simulink model "BasicModelTarget"  (Simulink 7.5)
settings: Solver=ode5  StartTime=0.0  StopTime=inf  FixedStep=sp/2  RelTol=1e-3
undefined symbols (not defined in the file or in its folder): AAz, BBz, sp
libraries: xpcnilib x10, xpclib x7
CloseFcn:
  | rtwprivate ssgencode ModelCloseRequest readecnoder
settings Model: Creator=Justin  LastModifiedBy=Justin  ExtModeArmWhenConnect=off  BufferReuse=off
settings DataIOCC: LimitDataPoints=off  MaxDataPoints=10000  SignalLoggingName=sigsOut
settings OptimizationCC: BlockReduction=off  BooleanDataType=off  OptimizeBlockIOStorage=off  BufferReuse=off  EnforceIntegerDowncast=off  ExpressionFolding=off  FoldNonRolledExpr=off  LocalBlockOutputs=off  InitFltsAndDblsToZero=on
settings DebuggingCC: SaveWithParameterizedLinksMsg=none  SignalResolutionControl=TryResolveAllWithWarning  SolverPrmCheckMsg=none  MultiTaskDSMMsg=warning  MultiTaskCondExecSysMsg=none  StrictBusMsg=None
settings HardwareCC: ProdIntDivRoundTo=Zero  ProdEndianess=LittleEndian  ProdHWDeviceType=Generic->32-bit x86 compatible  TargetHWDeviceType=32-bit Generic
settings RTWCC: SystemTargetFile=xpctarget.tlc  TemplateMakefile=xpc_default_tmf  Description=xPC Target  ProcessScript=xpctarget_make_rtw_hook  IncludeERTFirstTime=on  RTWCompilerOptimization=On
settings xpcTargetCC: TargetFcnLib=ansi_tfl_tmw.mat  TargetFunctionLibrary=ANSI_C  ERTCodeCoverageTool=None  ParMdlRefBuildCompliant=off  PortableWordSizes=off  xPCLoadParamSetFile=off

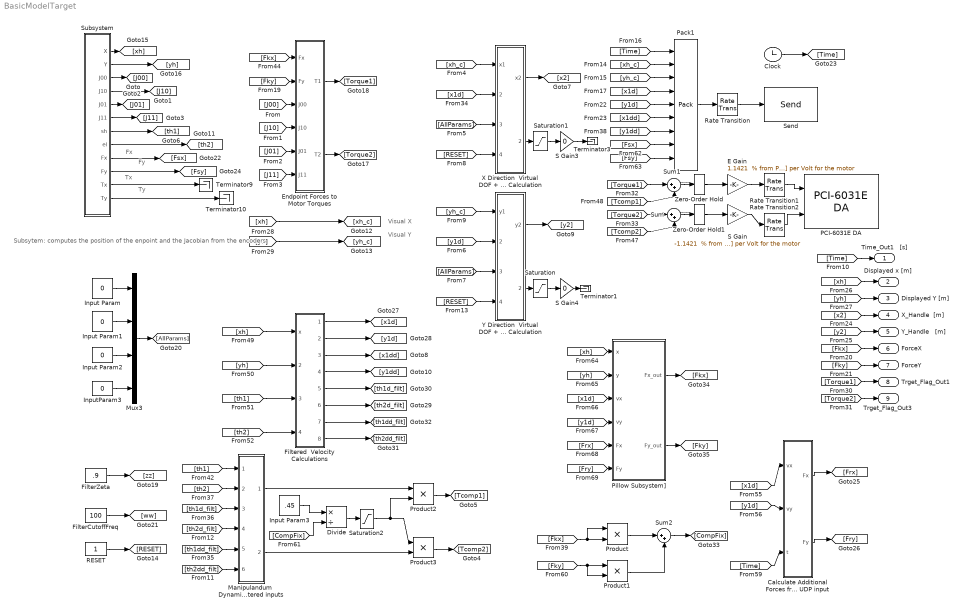
== system BasicModelTarget ==
  note: Subsytem:
      |  computes the position of the
      | enpoint and the Jacobian from
      | the encoders
  note: Ty
  note: Tx
  note: Fy
  note: Fx
  note: Visual X
  note: Visual Y
  " Calculate Additional Forces from UDP input" : Subsystem
  " Pillow Subsystem]" : Subsystem
  Clock : Clock
      settings: Decimation=10
  Divide : Product  Inputs=*/  OutDataType=fixdt(1, 16)  OutScaling=2^-10
  E Gain : Gain  Gain="1.1421  % from PCIO.H: [Nm] per Volt for the motor"  ParameterDataType=sfix(16)  ParameterScaling=2^0  OutDataType=sfix(16)  OutScaling=2^0  SaturateOnIntegerOverflow=on  OutDataTypeStr=Inherit: Same as input  ParamDataTypeStr=Inherit: Same as input
  Endpoint Forces to Motor Torques : Subsystem
  FilterCutoffFreq : Constant  Value=100  OutDataType=sfix(16)  OutScaling=2^0
  FilterZeta : Constant  Value=.9  OutDataType=sfix(16)  OutScaling=2^0
  Filtered  Velocity Calculations : Subsystem
  Input Param : Constant  Value=0  OutDataType=sfix(16)  OutScaling=2^0
  Input Param1 : Constant  Value=0  OutDataType=sfix(16)  OutScaling=2^0
  Input Param2 : Constant  Value=0  OutDataType=sfix(16)  OutScaling=2^0
  Input Param3 : Constant  Value=.45  OutDataType=sfix(16)  OutScaling=2^0
  InputParam3 : Constant  Value=0  OutDataType=sfix(16)  OutScaling=2^0
  Manipulandum  Dynamic Compensation: will function poorly with unfiltered inputs : Subsystem
  Mux3 : Mux
  PCI-6031E DA : xpcnilib/D//A/E Series/PCI-6031E DA  channel=[1 2]  range=[-10 -10]  reset=[1]  initValue=[0]  sampletime=sp  slot=-1
  Pack1 : xpclib/UDP/Pack  datatypes={'double','double','double','double','double','double','double','double','double'}  byteAlign=1
  Product{,1..3} (4 alike) : Product  OutDataType=fixdt(1, 16)  OutScaling=2^0  RndMeth=Zero
  RESET : Constant  OutDataType=sfix(16)  OutScaling=2^0
  Rate Transition : RateTransition
  Rate Transition1 : RateTransition
  Rate Transition2 : RateTransition
  S Gain : Gain  Gain="-1.1421  % from PCIO.H: [Nm] per Volt for the motor"  ParameterDataType=sfix(16)  ParameterScaling=2^0  OutDataType=sfix(16)  OutScaling=2^0  SaturateOnIntegerOverflow=on  OutDataTypeStr=Inherit: Same as input  ParamDataTypeStr=Inherit: Same as input
  S Gain3 : Gain  Gain=0  ParameterDataType=sfix(16)  ParameterScaling=2^0  OutDataType=sfix(16)  OutScaling=2^0  SaturateOnIntegerOverflow=on  OutDataTypeStr=Inherit: Same as input  ParamDataTypeStr=Inherit: Same as input
  S Gain4 : Gain  Gain=0  ParameterDataType=sfix(16)  ParameterScaling=2^0  OutDataType=sfix(16)  OutScaling=2^0  SaturateOnIntegerOverflow=on  OutDataTypeStr=Inherit: Same as input  ParamDataTypeStr=Inherit: Same as input
  Saturation : Saturate  UpperLimit=20  LowerLimit=-20
  Saturation1 : Saturate  UpperLimit=20  LowerLimit=-20
  Saturation2 : Saturate  UpperLimit=.4  LowerLimit=0
  Send : xpclib/UDP/Send  ipAddress=192.168.0.1  ipPort=25000  localPort=-1  vblLen=off  sampletime=sp*5
  Subsystem : Subsystem
  Sum : Sum  Inputs=|++  OutDataType=sfix(16)  OutScaling=2^0
  Sum1 : Sum  Inputs=|++  OutDataType=sfix(16)  OutScaling=2^0
  Sum2 : Sum  Inputs=|++  OutDataType=fixdt(1, 16)  OutScaling=2^0
  Terminator{1,3,9..10} (4 alike) : Terminator
  "X Direction  Virtual DOF + Endpoint Force Calculation " : Subsystem
  Y Direction  Virtual DOF + Endpoint Force Calculation : Subsystem
  Zero-Order Hold : ZeroOrderHold  SampleTime=sp*2
  Zero-Order Hold1 : ZeroOrderHold  SampleTime=sp*2
  Time_Out1   [s] : Outport  OutDataType=sfix(16)  OutScaling=2^0
  Displayed x [m] : Outport  Port=2  OutDataType=sfix(16)  OutScaling=2^0
  Displayed Y [m] : Outport  Port=3  OutDataType=sfix(16)  OutScaling=2^0
  X_Handle  [m] : Outport  Port=4  OutDataType=sfix(16)  OutScaling=2^0
  Y_Handle   [m] : Outport  Port=5  OutDataType=sfix(16)  OutScaling=2^0
  ForceX : Outport  Port=6  OutDataType=sfix(16)  OutScaling=2^0
  ForceY : Outport  Port=7  OutDataType=sfix(16)  OutScaling=2^0
  Trget_Flag_Out1 : Outport  Port=8  OutDataType=sfix(16)  OutScaling=2^0
  Trget_Flag_Out3 : Outport  Port=9  OutDataType=sfix(16)  OutScaling=2^0
  wires:
  Pack1/1 -> Rate Transition/1
  Clock/1 -> [Time]
  Subsystem/12(Ty) -> Terminator10/1
  Subsystem/11(Tx) -> Terminator9/1
  Subsystem/8(el) -> [th2]
  Subsystem/7(sh) -> [th1]
  E Gain/1 -> Rate Transition1/1
  S Gain/1 -> Rate Transition2/1
  Subsystem/10(Fy) -> [Fsy]
  [x2] -> X_Handle  [m]/1
  [xh] -> [xh_c]
  [yh] -> [yh_c]
  [y2] -> Y_Handle   [m]/1
  [Torque1] -> Trget_Flag_Out1/1
  [Torque2] -> Trget_Flag_Out3/1
  [Fkx] -> ForceX/1
  [Fky] -> ForceY/1
  [xh] -> Displayed x [m]/1
  [yh] -> Displayed Y [m]/1
  [Fky] -> Endpoint Forces to Motor Torques/2(Fy)
  [J00] -> Endpoint Forces to Motor Torques/3(J00)
  [J10] -> Endpoint Forces to Motor Torques/4(J10)
  [J01] -> Endpoint Forces to Motor Torques/5(J01)
  [J11] -> Endpoint Forces to Motor Torques/6(J11)
  Endpoint Forces to Motor Torques/1(T1) -> [Torque1]
  Endpoint Forces to Motor Torques/2(T2) -> [Torque2]
  [yh_c] -> Pack1/3
  [x1d] -> Pack1/4
  [y1d] -> Pack1/5
  [x1dd] -> Pack1/6
  "X Direction  Virtual DOF + Endpoint Force Calculation "/1(x2) -> [x2]
  [AllParams] -> "X Direction  Virtual DOF + Endpoint Force Calculation "/3(Params)
  [xh_c] -> "X Direction  Virtual DOF + Endpoint Force Calculation "/1(x1)
  Y Direction  Virtual DOF + Endpoint Force Calculation/2(Fky) -> Saturation/1
  Y Direction  Virtual DOF + Endpoint Force Calculation/1(y2) -> [y2]
  [RESET] -> Y Direction  Virtual DOF + Endpoint Force Calculation/4(Reset)
  [yh_c] -> Y Direction  Virtual DOF + Endpoint Force Calculation/1(y1)
  "X Direction  Virtual DOF + Endpoint Force Calculation "/2(Fkx) -> Saturation1/1
  Saturation1/1 -> S Gain3/1
  [y1dd] -> Pack1/7
  [x1d] -> "X Direction  Virtual DOF + Endpoint Force Calculation "/2(x1d)
  [RESET] -> "X Direction  Virtual DOF + Endpoint Force Calculation "/4(Reset)
  Mux3/1 -> [AllParams]
  Input Param/1 -> Mux3/1
  Input Param1/1 -> Mux3/2
  Input Param2/1 -> Mux3/3
  InputParam3/1 -> Mux3/4
  [y1d] -> Y Direction  Virtual DOF + Endpoint Force Calculation/2(y1d)
  [AllParams] -> Y Direction  Virtual DOF + Endpoint Force Calculation/3(Params)
  Subsystem/1(X) -> [xh]
  Subsystem/2(Y) -> [yh]
  Subsystem/3(J00) -> [J00]
  Subsystem/4(J10) -> [J10]
  Subsystem/5(J01) -> [J01]
  Subsystem/6(J11) -> [J11]
  [Time] -> Time_Out1   [s]/1
  [th1] -> Manipulandum  Dynamic Compensation: will function poorly with unfiltered inputs/1(th1)
  [th2] -> Manipulandum  Dynamic Compensation: will function poorly with unfiltered inputs/2(th2)
  [th1d_filt] -> Manipulandum  Dynamic Compensation: will function poorly with unfiltered inputs/3(th1d)
  [th2d_filt] -> Manipulandum  Dynamic Compensation: will function poorly with unfiltered inputs/4(th2d)
  [th1dd_filt] -> Manipulandum  Dynamic Compensation: will function poorly with unfiltered inputs/5(th1dd)
  [th2dd_filt] -> Manipulandum  Dynamic Compensation: will function poorly with unfiltered inputs/6(th2dd)
  [Torque2] -> Sum/1
  [Tcomp2] -> Sum/2
  Sum/1 -> Zero-Order Hold1/1
  [Tcomp1] -> Sum1/2
  [Torque1] -> Sum1/1
  Sum1/1 -> Zero-Order Hold/1
  Saturation/1 -> S Gain4/1
  Subsystem/9(Fx) -> [Fsx]
  Zero-Order Hold/1 -> E Gain/1
  Zero-Order Hold1/1 -> S Gain/1
  FilterZeta/1 -> [zz]
  FilterCutoffFreq/1 -> [ww]
  RESET/1 -> [RESET]
  S Gain4/1 -> Terminator1/1
  S Gain3/1 -> Terminator3/1
  Rate Transition/1 -> Send/1
  Rate Transition1/1 -> PCI-6031E DA/1
  Rate Transition2/1 -> PCI-6031E DA/2
  [Fkx] -> Endpoint Forces to Motor Torques/1(Fx)
  [Time] -> Pack1/1
  [xh_c] -> Pack1/2
  [Fkx] -> Product/1, Product/2
  [Fky] -> Product1/1, Product1/2
  Product/1 -> Sum2/1
  Product1/1 -> Sum2/2
  Manipulandum  Dynamic Compensation: will function poorly with unfiltered inputs/1(Tc1) -> Product2/1
  Manipulandum  Dynamic Compensation: will function poorly with unfiltered inputs/2(Tc2) -> Product3/2
  Product3/1 -> [Tcomp2]
  Product2/1 -> [Tcomp1]
  Input Param3/1 -> Divide/1
  [CompFix] -> Divide/2
  Divide/1 -> Saturation2/1
  Saturation2/1 -> Product2/2, Product3/1
  Sum2/1 -> [CompFix]
  [Fsx] -> Pack1/8
  [Fsy] -> Pack1/9
  [xh] -> " Pillow Subsystem]"/1(x)
  [yh] -> " Pillow Subsystem]"/2(y)
  [x1d] -> " Pillow Subsystem]"/3(vx)
  [y1d] -> " Pillow Subsystem]"/4(vy)
  [Frx] -> " Pillow Subsystem]"/5(Fx)
  [Fry] -> " Pillow Subsystem]"/6(Fy)
  " Pillow Subsystem]"/1(Fx_out) -> [Fkx]
  " Pillow Subsystem]"/2(Fy_out) -> [Fky]
  Filtered  Velocity Calculations/1(Out1) -> [x1d]
  Filtered  Velocity Calculations/2(Out2) -> [y1d]
  [xh] -> Filtered  Velocity Calculations/1(x)
  [yh] -> Filtered  Velocity Calculations/2(In2)
  [th1] -> Filtered  Velocity Calculations/3(In3)
  [th2] -> Filtered  Velocity Calculations/4(In4)
  Filtered  Velocity Calculations/3(xdd) -> [x1dd]
  Filtered  Velocity Calculations/4(Out4) -> [y1dd]
  Filtered  Velocity Calculations/5(Out5) -> [th1d_filt]
  Filtered  Velocity Calculations/6(Out6) -> [th2d_filt]
  Filtered  Velocity Calculations/7(Out7) -> [th1dd_filt]
  Filtered  Velocity Calculations/8(Out8) -> [th2dd_filt]
  [x1d] -> " Calculate Additional Forces from UDP input"/1(vx)
  [y1d] -> " Calculate Additional Forces from UDP input"/2(vy)
  " Calculate Additional Forces from UDP input"/1(Fx) -> [Frx]
  " Calculate Additional Forces from UDP input"/2(Fy) -> [Fry]
  [Time] -> " Calculate Additional Forces from UDP input"/3(t)

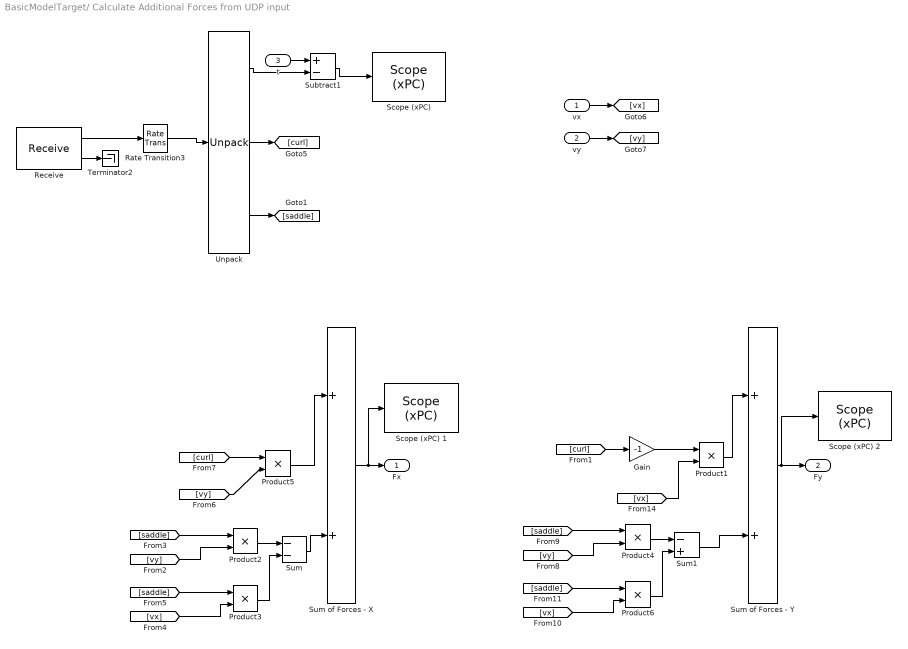
== system BasicModelTarget/ Calculate Additional Forces from UDP input ==
  vx : Inport  OutDataType=fixdt(1, 16)  OutScaling=2^0
  vy : Inport  Port=2  OutDataType=fixdt(1, 16)  OutScaling=2^0
  t : Inport  Port=3  OutDataType=fixdt(1, 16)  OutScaling=2^0
  Gain : Gain  Gain=-1  ParameterDataType=fixdt(1, 16)  ParameterScaling=2^0  OutDataType=fixdt(1, 16)  OutScaling=2^0
  Product{1..6} (6 alike) : Product  OutDataType=fixdt(1, 16)  OutScaling=2^0  RndMeth=Zero
  Rate Transition3 : RateTransition
  Receive : xpclib/UDP/Receive  ipAddress=0.0.0.0  ipPort=25000  width=8*3  vblLen=off  sampletime=sp*5
  "Scope (xPC) " : xpclib/Misc./Scope (xPC)   SystemSampleTime=-1  scopeno=4  scopetype=Target  autostart=on  viewmode=Numerical  formatstr='%15.6f'  grid=on  ylimits=[-6,6]  nosamples=250  noprepostsamples=0  interleave=1  triggermode=FreeRun  triggersignal=1  triggerlevel=0.0  triggerslope=Either  triggerscope=1  triggersample=0  filename=data.dat  mode=Lazy  writesize=512  autorestart=off  dynamicfilemode=off  maxwritefilesize=512*1024^2
  Scope (xPC) 1 : xpclib/Misc./Scope (xPC)   SystemSampleTime=-1  scopeno=1  scopetype=Target  autostart=on  viewmode=Graphical redraw  formatstr='%15.6f'  grid=on  ylimits=[-6,6]  nosamples=250  noprepostsamples=0  interleave=1  triggermode=FreeRun  triggersignal=1  triggerlevel=0.0  triggerslope=Either  triggerscope=1  triggersample=0  filename=data.dat  mode=Lazy  writesize=512  autorestart=off  dynamicfilemode=off  maxwritefilesize=512*1024^2
  Scope (xPC) 2 : xpclib/Misc./Scope (xPC)   SystemSampleTime=-1  scopeno=2  scopetype=Target  autostart=on  viewmode=Graphical redraw  formatstr='%15.6f'  grid=on  ylimits=[-6,6]  nosamples=250  noprepostsamples=0  interleave=1  triggermode=FreeRun  triggersignal=1  triggerlevel=0.0  triggerslope=Either  triggerscope=1  triggersample=0  filename=data.dat  mode=Lazy  writesize=512  autorestart=off  dynamicfilemode=off  maxwritefilesize=512*1024^2
  Subtract1 : Sum  Inputs=+-  OutDataType=fixdt(1, 16)  OutScaling=2^-10
  Sum : Sum  Inputs=--  OutDataType=fixdt(1, 16)  OutScaling=2^-10
  Sum of Forces - X : Sum  OutDataType=fixdt(1, 16)  OutScaling=2^-10
  Sum of Forces - Y : Sum  OutDataType=fixdt(1, 16)  OutScaling=2^-10
  Sum1 : Sum  Inputs=-+  OutDataType=fixdt(1, 16)  OutScaling=2^-10
  Terminator2 : Terminator
  Unpack : xpclib/UDP/Unpack  dimensions={1,1,1}  datatypes={'double','double','double'}  byteAlign=1
  Fx : Outport  OutDataType=fixdt(1, 16)  OutScaling=2^0
  Fy : Outport  Port=2  OutDataType=fixdt(1, 16)  OutScaling=2^0
  wires:
  Sum1/1 -> Sum of Forces - Y/2
  [vy] -> Product4/2
  Product6/1 -> Sum1/2
  [vx] -> Product6/2
  [saddle] -> Product6/1
  Product4/1 -> Sum1/1
  [saddle] -> Product4/1
  [vy] -> Product2/2
  Product3/1 -> Sum/2
  [vx] -> Product3/2
  [saddle] -> Product3/1
  Sum/1 -> Sum of Forces - X/2
  Product2/1 -> Sum/1
  [saddle] -> Product2/1
  Unpack/3 -> [saddle]
  Product1/1 -> Sum of Forces - Y/1
  [curl] -> Gain/1
  Gain/1 -> Product1/1
  [vx] -> Product1/2
  Product5/1 -> Sum of Forces - X/1
  Unpack/2 -> [curl]
  Unpack/1 -> Subtract1/2
  Sum of Forces - Y/1 -> Scope (xPC) 2/1, Fy/1
  [vy] -> Product5/2
  [curl] -> Product5/1
  vy/1 -> [vy]
  vx/1 -> [vx]
  Sum of Forces - X/1 -> Scope (xPC) 1/1, Fx/1
  t/1 -> Subtract1/1
  Rate Transition3/1 -> Unpack/1
  Receive/1 -> Rate Transition3/1
  Subtract1/1 -> "Scope (xPC) "/1
  Receive/2 -> Terminator2/1

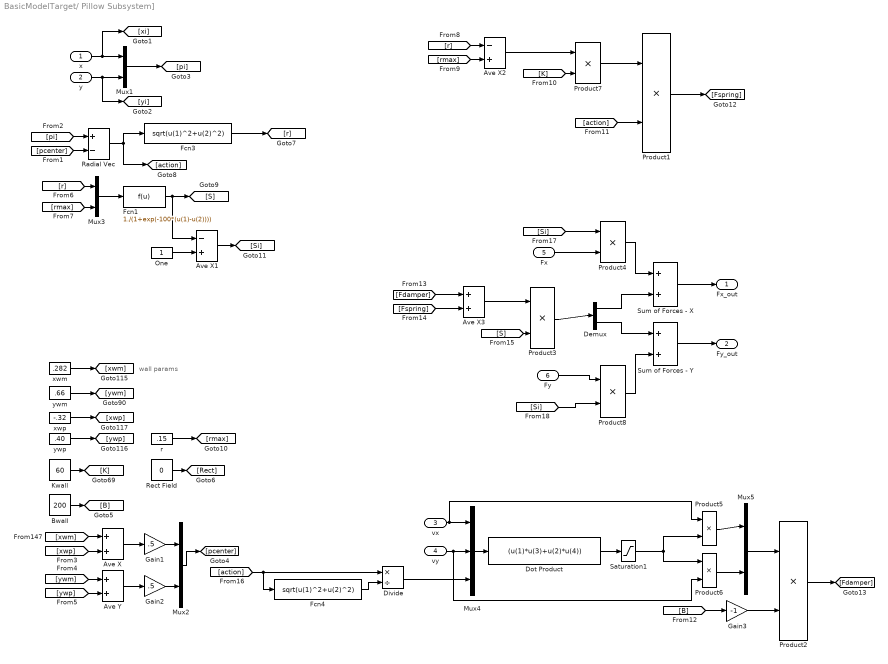
== system BasicModelTarget/ Pillow Subsystem] ==
  note: wall params
  x : Inport  OutDataType=fixdt(1, 16)  OutScaling=2^0
  y : Inport  Port=2  OutDataType=fixdt(1, 16)  OutScaling=2^0
  vx : Inport  Port=3  OutDataType=fixdt(1, 16)  OutScaling=2^0
  vy : Inport  Port=4  OutDataType=fixdt(1, 16)  OutScaling=2^0
  Fx : Inport  Port=5  OutDataType=fixdt(1, 16)  OutScaling=2^0
  Fy : Inport  Port=6  OutDataType=fixdt(1, 16)  OutScaling=2^0
  Ave X : Sum  OutDataType=fixdt(1, 16)  OutScaling=2^-10
  Ave X1 : Sum  Inputs=-+  OutDataType=fixdt(1, 16)  OutScaling=2^-10
  Ave X2 : Sum  Inputs=-+  OutDataType=fixdt(1, 16)  OutScaling=2^-10
  Ave X3 : Sum  OutDataType=fixdt(1, 16)  OutScaling=2^-10
  Ave Y : Sum  OutDataType=fixdt(1, 16)  OutScaling=2^-10
  Bwall : Constant  Value=200  OutDataType=sfix(16)  OutScaling=2^0
  Demux : Demux  Outputs=2
  Divide : Product  Inputs=*/  OutDataType=fixdt(1, 16)  OutScaling=2^-10
  Dot Product : Fcn  Expr=(u(1)*u(3)+u(2)*u(4))
  Fcn1 : Fcn  Expr=1./(1+exp(-100*(u(1)-u(2))))
  Fcn3 : Fcn  Expr=sqrt(u(1)^2+u(2)^2)
  Fcn4 : Fcn  Expr=sqrt(u(1)^2+u(2)^2)
  Gain1 : Gain  Gain=.5  ParameterDataType=fixdt(1, 16)  ParameterScaling=2^0  OutDataType=fixdt(1, 16)  OutScaling=2^0
  Gain2 : Gain  Gain=.5  ParameterDataType=fixdt(1, 16)  ParameterScaling=2^0  OutDataType=fixdt(1, 16)  OutScaling=2^0
  Gain3 : Gain  Gain=-1  ParameterDataType=fixdt(1, 16)  ParameterScaling=2^0  OutDataType=fixdt(1, 16)  OutScaling=2^0
  Kwall : Constant  Value=60  OutDataType=sfix(16)  OutScaling=2^0
  Mux{1..3,5} (4 alike) : Mux  Inputs=2
  Mux4 : Mux  Inputs=3
  One : Constant  OutDataType=sfix(16)  OutScaling=2^0
  Product{1..8} (8 alike) : Product  OutDataType=sfix(16)  OutScaling=2^0  RndMeth=Zero
  Radial Vec : Sum  Inputs=+-  OutDataType=fixdt(1, 16)  OutScaling=2^-10
  Rect Field : Constant  Value=0  OutDataType=sfix(16)  OutScaling=2^0
  Saturation1 : Saturate  UpperLimit=inf  LowerLimit=0
  Sum of Forces - X : Sum  OutDataType=fixdt(1, 16)  OutScaling=2^-10
  Sum of Forces - Y : Sum  OutDataType=fixdt(1, 16)  OutScaling=2^-10
  r : Constant  Value=.15  OutDataType=sfix(16)  OutScaling=2^0
  xwm : Constant  Value=.282  OutDataType=sfix(16)  OutScaling=2^0
  xwp : Constant  Value=-.32  OutDataType=sfix(16)  OutScaling=2^0
  ywm : Constant  Value=.66  OutDataType=sfix(16)  OutScaling=2^0
  ywp : Constant  Value=.40  OutDataType=sfix(16)  OutScaling=2^0
  Fx_out : Outport  OutDataType=fixdt(1, 16)  OutScaling=2^0
  Fy_out : Outport  Port=2  OutDataType=fixdt(1, 16)  OutScaling=2^0
  wires:
  ywp/1 -> [ywp]
  xwp/1 -> [xwp]
  xwm/1 -> [xwm]
  ywm/1 -> [ywm]
  Kwall/1 -> [K]
  Sum of Forces - X/1 -> Fx_out/1
  Sum of Forces - Y/1 -> Fy_out/1
  x/1 -> Mux1/1, [xi]
  y/1 -> Mux1/2, [yi]
  Mux1/1 -> [pi]
  Mux2/1 -> [pcenter]
  [xwm] -> Ave X/1
  [xwp] -> Ave X/2
  [ywp] -> Ave Y/2
  [ywm] -> Ave Y/1
  Ave X/1 -> Gain1/1
  Gain1/1 -> Mux2/1
  Ave Y/1 -> Gain2/1
  Gain2/1 -> Mux2/2
  Bwall/1 -> [B]
  Rect Field/1 -> [Rect]
  [pi] -> Radial Vec/1
  [pcenter] -> Radial Vec/2
  Radial Vec/1 -> Fcn3/1, [action]
  Fcn3/1 -> [r]
  r/1 -> [rmax]
  [r] -> Mux3/1
  [rmax] -> Mux3/2
  Mux3/1 -> Fcn1/1
  Fcn1/1 -> Ave X1/1, [S]
  One/1 -> Ave X1/2
  Ave X1/1 -> [Si]
  [r] -> Ave X2/1
  [rmax] -> Ave X2/2
  Ave X2/1 -> Product7/1
  [K] -> Product7/2
  Product7/1 -> Product1/1
  [action] -> Product1/2
  Product1/1 -> [Fspring]
  vx/1 -> Mux4/1, Product5/1
  vy/1 -> Mux4/2, Product6/2
  Product2/1 -> [Fdamper]
  [Fdamper] -> Ave X3/1
  [Fspring] -> Ave X3/2
  Ave X3/1 -> Product3/1
  [S] -> Product3/2
  Product3/1 -> Demux/1
  Product4/1 -> Sum of Forces - X/1
  Demux/1 -> Sum of Forces - X/2
  Demux/2 -> Sum of Forces - Y/1
  Fy/1 -> Product8/1
  [Si] -> Product4/1
  Fx/1 -> Product4/2
  Mux4/1 -> Dot Product/1
  Mux5/1 -> Product2/1
  [action] -> Fcn4/1, Divide/1
  Divide/1 -> Mux4/3
  Fcn4/1 -> Divide/2
  [B] -> Gain3/1
  Gain3/1 -> Product2/2
  Dot Product/1 -> Saturation1/1
  Product5/1 -> Mux5/1
  Product6/1 -> Mux5/2
  Saturation1/1 -> Product5/2, Product6/1
  [Si] -> Product8/2
  Product8/1 -> Sum of Forces - Y/2

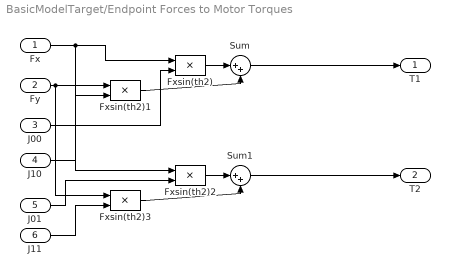
== system BasicModelTarget/Endpoint Forces to Motor Torques ==
  Fx : Inport  OutDataType=sfix(16)  OutScaling=2^0
  Fy : Inport  Port=2  OutDataType=sfix(16)  OutScaling=2^0
  J00 : Inport  Port=3  OutDataType=sfix(16)  OutScaling=2^0
  J10 : Inport  Port=4  OutDataType=sfix(16)  OutScaling=2^0
  J01 : Inport  Port=5  OutDataType=sfix(16)  OutScaling=2^0
  J11 : Inport  Port=6  OutDataType=sfix(16)  OutScaling=2^0
  Fxsin(th2){,1..3} (4 alike) : Product  OutDataType=sfix(16)  OutScaling=2^0  SaturateOnIntegerOverflow=on  OutDataTypeStr=Inherit: Same as first input
  Sum : Sum  Inputs=|++  OutDataType=sfix(16)  OutScaling=2^0  SaturateOnIntegerOverflow=on  InputSameDT=on  OutDataTypeStr=Inherit: Same as first input
  Sum1 : Sum  Inputs=|++  OutDataType=sfix(16)  OutScaling=2^0  SaturateOnIntegerOverflow=on  InputSameDT=on  OutDataTypeStr=Inherit: Same as first input
  T1 : Outport  OutDataType=sfix(16)  OutScaling=2^0
  T2 : Outport  Port=2  OutDataType=sfix(16)  OutScaling=2^0
  wires:
  Sum/1 -> T1/1
  Fxsin(th2)/1 -> Sum/1
  Fxsin(th2)1/1 -> Sum/2
  Fxsin(th2)2/1 -> Sum1/1
  Fxsin(th2)3/1 -> Sum1/2
  Sum1/1 -> T2/1
  Fx/1 -> Fxsin(th2)/1, Fxsin(th2)2/1
  Fy/1 -> Fxsin(th2)1/1, Fxsin(th2)3/1
  J11/1 -> Fxsin(th2)3/2
  J01/1 -> Fxsin(th2)2/2
  J10/1 -> Fxsin(th2)1/2
  J00/1 -> Fxsin(th2)/2

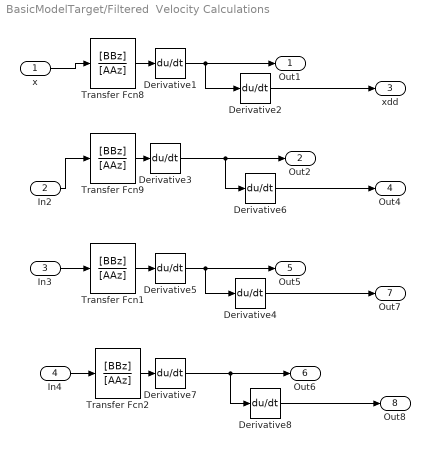
== system BasicModelTarget/Filtered  Velocity Calculations ==
  x : Inport  OutDataType=sfix(16)  OutScaling=2^0
  In2 : Inport  Port=2  OutDataType=sfix(16)  OutScaling=2^0
  In3 : Inport  Port=3  OutDataType=sfix(16)  OutScaling=2^0
  In4 : Inport  Port=4  OutDataType=sfix(16)  OutScaling=2^0
  Derivative{1..8} (8 alike) : Derivative
  Transfer Fcn{1..2,8..9} (4 alike) : TransferFcn  Numerator=[BBz]  Denominator=[AAz]
  Out1 : Outport  OutDataType=sfix(16)  OutScaling=2^0
  Out2 : Outport  Port=2  OutDataType=sfix(16)  OutScaling=2^0
  xdd : Outport  Port=3  OutDataType=sfix(16)  OutScaling=2^0
  Out4 : Outport  Port=4  OutDataType=sfix(16)  OutScaling=2^0
  Out5 : Outport  Port=5  OutDataType=sfix(16)  OutScaling=2^0
  Out6 : Outport  Port=6  OutDataType=sfix(16)  OutScaling=2^0
  Out7 : Outport  Port=7  OutDataType=sfix(16)  OutScaling=2^0
  Out8 : Outport  Port=8  OutDataType=sfix(16)  OutScaling=2^0
  wires:
  x/1 -> Transfer Fcn8/1
  Derivative1/1 -> Out1/1, Derivative2/1
  Derivative3/1 -> Out2/1, Derivative6/1
  In2/1 -> Transfer Fcn9/1
  Transfer Fcn8/1 -> Derivative1/1
  Transfer Fcn9/1 -> Derivative3/1
  In3/1 -> Transfer Fcn1/1
  In4/1 -> Transfer Fcn2/1
  Derivative2/1 -> xdd/1
  Derivative6/1 -> Out4/1
  Derivative5/1 -> Out5/1, Derivative4/1
  Derivative7/1 -> Out6/1, Derivative8/1
  Transfer Fcn1/1 -> Derivative5/1
  Transfer Fcn2/1 -> Derivative7/1
  Derivative4/1 -> Out7/1
  Derivative8/1 -> Out8/1

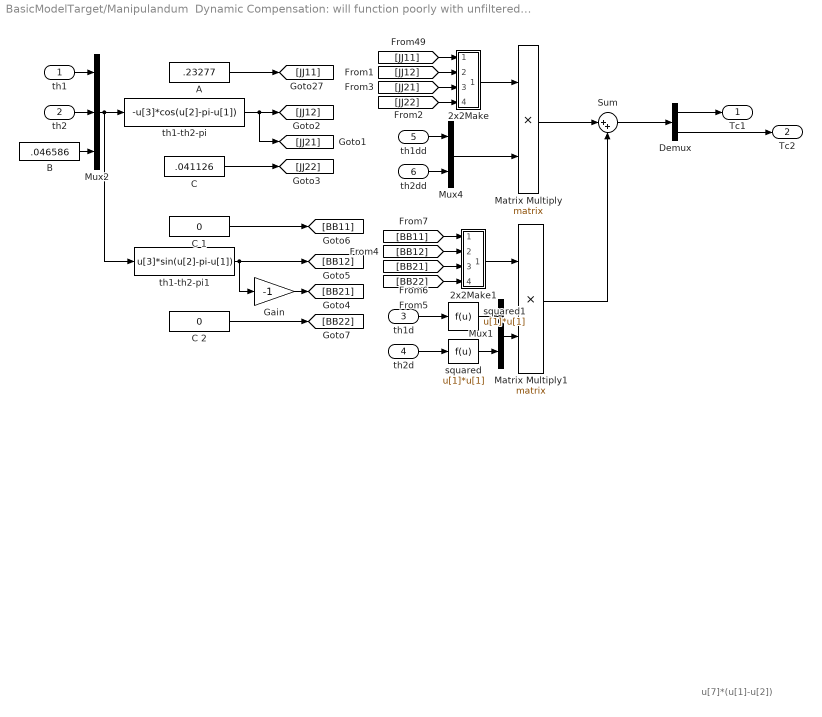
== system BasicModelTarget/Manipulandum  Dynamic Compensation: will function poorly with unfiltered inputs ==
  note: u[7]*(u[1]-u[2])
  th1 : Inport  OutDataType=sfix(16)  OutScaling=2^0
  th2 : Inport  Port=2  OutDataType=sfix(16)  OutScaling=2^0
  th1d : Inport  Port=3  OutDataType=sfix(16)  OutScaling=2^0
  th2d : Inport  Port=4  OutDataType=sfix(16)  OutScaling=2^0
  th1dd : Inport  Port=5  OutDataType=sfix(16)  OutScaling=2^0
  th2dd : Inport  Port=6  OutDataType=sfix(16)  OutScaling=2^0
  2x2Make : Subsystem
  2x2Make1 : Subsystem
  A : Constant  Value=.23277  OutDataType=sfix(16)  OutScaling=2^0
  B : Constant  Value=.046586  OutDataType=sfix(16)  OutScaling=2^0
  "C " : Constant  Value=.041126  OutDataType=sfix(16)  OutScaling=2^0
  C 1 : Constant  Value=0  OutDataType=sfix(16)  OutScaling=2^0
  C 2 : Constant  Value=0  OutDataType=sfix(16)  OutScaling=2^0
  Demux : Demux  Outputs=2
  Gain : Gain  Gain=-1  ParameterDataType=sfix(16)  ParameterScaling=2^0  OutDataType=sfix(16)  OutScaling=2^0
  Matrix Multiply : Product  Multiplication=Matrix(*)  OutDataType=sfix(16)  OutScaling=2^0
  Matrix Multiply1 : Product  Multiplication=Matrix(*)  OutDataType=sfix(16)  OutScaling=2^0
  Mux1 : Mux  Inputs=2
  Mux2 : Mux  Inputs=3
  Mux4 : Mux  Inputs=2
  Sum : Sum  Inputs=|++  OutDataType=sfix(16)  OutScaling=2^0
  squared : Fcn  Expr=u[1]*u[1]
  squared1 : Fcn  Expr=u[1]*u[1]
  th1-th2-pi : Fcn  Expr=-u[3]*cos(u[2]-pi-u[1])
  th1-th2-pi1 : Fcn  Expr=u[3]*sin(u[2]-pi-u[1])
  Tc1 : Outport  OutDataType=sfix(16)  OutScaling=2^0
  Tc2 : Outport  Port=2  OutDataType=sfix(16)  OutScaling=2^0
  wires:
  th2d/1 -> squared/1
  th1dd/1 -> Mux4/1
  th2dd/1 -> Mux4/2
  th2/1 -> Mux2/2
  th1/1 -> Mux2/1
  Mux2/1 -> th1-th2-pi/1, th1-th2-pi1/1
  A/1 -> [JJ11]
  B/1 -> Mux2/3
  th1-th2-pi/1 -> [JJ12], [JJ21]
  "C "/1 -> [JJ22]
  [JJ11] -> 2x2Make/1(In1)
  [JJ12] -> 2x2Make/2(In2)
  [JJ21] -> 2x2Make/3(In3)
  [JJ22] -> 2x2Make/4(In4)
  2x2Make/1(Out1) -> Matrix Multiply/1
  Mux4/1 -> Matrix Multiply/2
  [BB11] -> 2x2Make1/1(In1)
  [BB12] -> 2x2Make1/2(In2)
  [BB21] -> 2x2Make1/3(In3)
  [BB22] -> 2x2Make1/4(In4)
  th1d/1 -> squared1/1
  2x2Make1/1(Out1) -> Matrix Multiply1/1
  Mux1/1 -> Matrix Multiply1/2
  C 2/1 -> [BB22]
  th1-th2-pi1/1 -> [BB12], Gain/1
  C 1/1 -> [BB11]
  Gain/1 -> [BB21]
  Matrix Multiply/1 -> Sum/1
  Matrix Multiply1/1 -> Sum/2
  squared/1 -> Mux1/2
  squared1/1 -> Mux1/1
  Sum/1 -> Demux/1
  Demux/1 -> Tc1/1
  Demux/2 -> Tc2/1

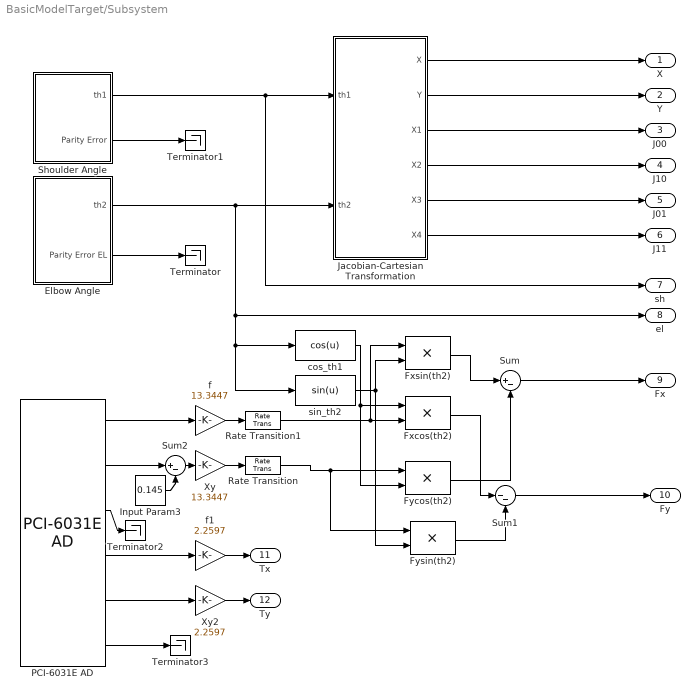
== system BasicModelTarget/Subsystem ==
  Elbow Angle : Subsystem
  Fxcos(th2) : Product  OutDataType=sfix(16)  OutScaling=2^0  SaturateOnIntegerOverflow=on  OutDataTypeStr=Inherit: Same as first input
  Fxsin(th2) : Product  OutDataType=sfix(16)  OutScaling=2^0  SaturateOnIntegerOverflow=on  OutDataTypeStr=Inherit: Same as first input
  Fycos(th2) : Product  OutDataType=sfix(16)  OutScaling=2^0  SaturateOnIntegerOverflow=on  OutDataTypeStr=Inherit: Same as first input
  Fysin(th2) : Product  OutDataType=sfix(16)  OutScaling=2^0  SaturateOnIntegerOverflow=on  OutDataTypeStr=Inherit: Same as first input
  Input Param3 : Constant  Value=0.145  OutDataType=sfix(16)  OutScaling=2^0
  Jacobian-Cartesian Transformation : Subsystem
  PCI-6031E AD : xpcnilib/A//D/E Series/PCI-6031E AD  channel=[1, 2, 3, 4, 5, 6]  range=[-5, -5, -5, -5, -5, -5]  coupling=[2, 2, 2, 2, 2, 2]  sampletime=sp  slot=-1
  Rate Transition : RateTransition
  Rate Transition1 : RateTransition
  Shoulder Angle : Subsystem
  Sum : Sum  Inputs=|+-  OutDataType=sfix(16)  OutScaling=2^0  SaturateOnIntegerOverflow=on  InputSameDT=on  OutDataTypeStr=Inherit: Same as first input
  Sum1 : Sum  Inputs=|--  OutDataType=sfix(16)  OutScaling=2^0  SaturateOnIntegerOverflow=on  InputSameDT=on  OutDataTypeStr=Inherit: Same as first input
  Sum2 : Sum  Inputs=|+-  OutDataType=sfix(16)  OutScaling=2^0  SaturateOnIntegerOverflow=on  InputSameDT=on  OutDataTypeStr=Inherit: Same as first input
  Terminator{,1..3} (4 alike) : Terminator
  Xy : Gain  Gain=13.3447  ParameterDataType=sfix(16)  ParameterScaling=2^0  OutDataType=sfix(16)  OutScaling=2^0  SaturateOnIntegerOverflow=on  OutDataTypeStr=Inherit: Same as input  ParamDataTypeStr=Inherit: Same as input
  Xy2 : Gain  Gain=2.2597  ParameterDataType=sfix(16)  ParameterScaling=2^0  OutDataType=sfix(16)  OutScaling=2^0  SaturateOnIntegerOverflow=on  OutDataTypeStr=Inherit: Same as input  ParamDataTypeStr=Inherit: Same as input
  cos_th1 : Fcn  Expr=cos(u)
  f : Gain  Gain=13.3447  ParameterDataType=sfix(16)  ParameterScaling=2^0  OutDataType=sfix(16)  OutScaling=2^0  SaturateOnIntegerOverflow=on  OutDataTypeStr=Inherit: Same as input  ParamDataTypeStr=Inherit: Same as input
  f1 : Gain  Gain=2.2597  ParameterDataType=sfix(16)  ParameterScaling=2^0  OutDataType=sfix(16)  OutScaling=2^0  SaturateOnIntegerOverflow=on  OutDataTypeStr=Inherit: Same as input  ParamDataTypeStr=Inherit: Same as input
  sin_th2 : Fcn  Expr=sin(u)
  X : Outport  OutDataType=sfix(16)  OutScaling=2^0
  Y : Outport  Port=2  OutDataType=sfix(16)  OutScaling=2^0
  J00 : Outport  Port=3  OutDataType=sfix(16)  OutScaling=2^0
  J10 : Outport  Port=4  OutDataType=sfix(16)  OutScaling=2^0
  J01 : Outport  Port=5  OutDataType=sfix(16)  OutScaling=2^0
  J11 : Outport  Port=6  OutDataType=sfix(16)  OutScaling=2^0
  sh : Outport  Port=7  OutDataType=sfix(16)  OutScaling=2^0
  el : Outport  Port=8  OutDataType=sfix(16)  OutScaling=2^0
  Fx : Outport  Port=9  OutDataType=sfix(16)  OutScaling=2^0
  Fy : Outport  Port=10  OutDataType=sfix(16)  OutScaling=2^0
  Tx : Outport  Port=11  OutDataType=sfix(16)  OutScaling=2^0
  Ty : Outport  Port=12  OutDataType=sfix(16)  OutScaling=2^0
  wires:
  Shoulder Angle/1(th1) -> Jacobian-Cartesian Transformation/1(th1), sh/1
  Elbow Angle/1(th2) -> Jacobian-Cartesian Transformation/2(th2), el/1, sin_th2/1, cos_th1/1
  Jacobian-Cartesian Transformation/1(X) -> X/1
  Jacobian-Cartesian Transformation/2(Y) -> Y/1
  Elbow Angle/2(Parity Error EL) -> Terminator/1
  Shoulder Angle/2(Parity Error) -> Terminator1/1
  Jacobian-Cartesian Transformation/3(X1) -> J00/1
  Jacobian-Cartesian Transformation/4(X2) -> J10/1
  Jacobian-Cartesian Transformation/5(X3) -> J01/1
  Jacobian-Cartesian Transformation/6(X4) -> J11/1
  sin_th2/1 -> Fxsin(th2)/2, Fysin(th2)/2
  cos_th1/1 -> Fxcos(th2)/1, Fycos(th2)/2
  Fxsin(th2)/1 -> Sum/1
  Sum/1 -> Fx/1
  Fysin(th2)/1 -> Sum1/2
  Sum1/1 -> Fy/1
  Fycos(th2)/1 -> Sum/2
  Fxcos(th2)/1 -> Sum1/1
  Xy2/1 -> Ty/1
  PCI-6031E AD/5 -> Xy2/1
  f1/1 -> Tx/1
  PCI-6031E AD/4 -> f1/1
  PCI-6031E AD/1 -> f/1
  f/1 -> Rate Transition1/1
  Xy/1 -> Rate Transition/1
  Rate Transition/1 -> Fycos(th2)/1, Fysin(th2)/1
  Rate Transition1/1 -> Fxsin(th2)/1, Fxcos(th2)/2
  PCI-6031E AD/3 -> Terminator2/1
  PCI-6031E AD/6 -> Terminator3/1
  PCI-6031E AD/2 -> Sum2/1
  Sum2/1 -> Xy/1
  Input Param3/1 -> Sum2/2

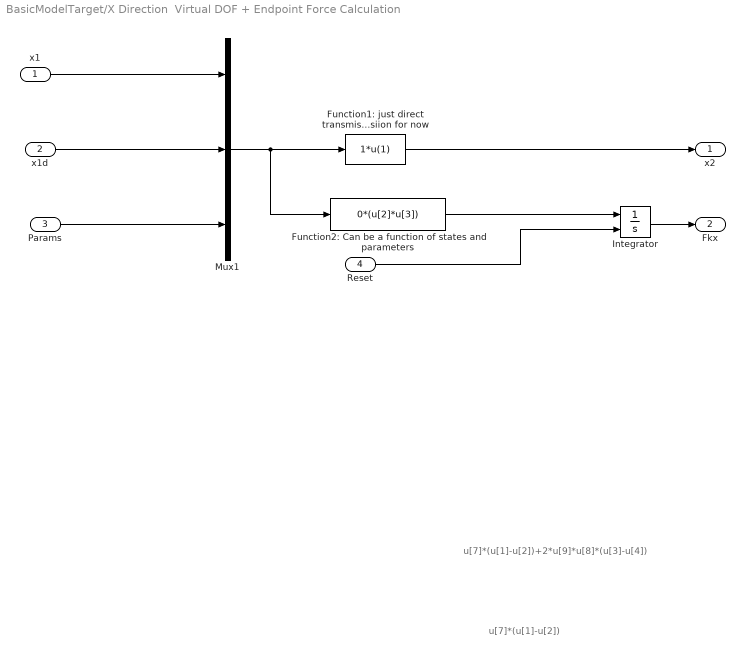
== system BasicModelTarget/X Direction  Virtual DOF + Endpoint Force Calculation  ==
  note: u[7]*(u[1]-u[2])
  note: u[7]*(u[1]-u[2])+2*u[9]*u[8]*(u[3]-u[4])
  x1 : Inport  OutDataType=sfix(16)  OutScaling=2^0
  x1d : Inport  Port=2  OutDataType=sfix(16)  OutScaling=2^0
  Params : Inport  Port=3  OutDataType=sfix(16)  OutScaling=2^0
  Reset : Inport  Port=4  OutDataType=sfix(16)  OutScaling=2^0
  Function1: just direct transmissiion for now : Fcn  Expr=1*u(1)
  Function2: Can be a function of states and parameters : Fcn  Expr=0*(u[2]*u[3])
  Integrator : Integrator  ExternalReset=either
  Mux1 : Mux  Inputs=3
  x2 : Outport  OutDataType=sfix(16)  OutScaling=2^0
  Fkx : Outport  Port=2  OutDataType=sfix(16)  OutScaling=2^0
  wires:
  Function1: just direct transmissiion for now/1 -> x2/1
  Mux1/1 -> Function2: Can be a function of states and parameters/1, Function1: just direct transmissiion for now/1
  x1/1 -> Mux1/1
  Function2: Can be a function of states and parameters/1 -> Integrator/1
  Integrator/1 -> Fkx/1
  Reset/1 -> Integrator/2
  Params/1 -> Mux1/3
  x1d/1 -> Mux1/2

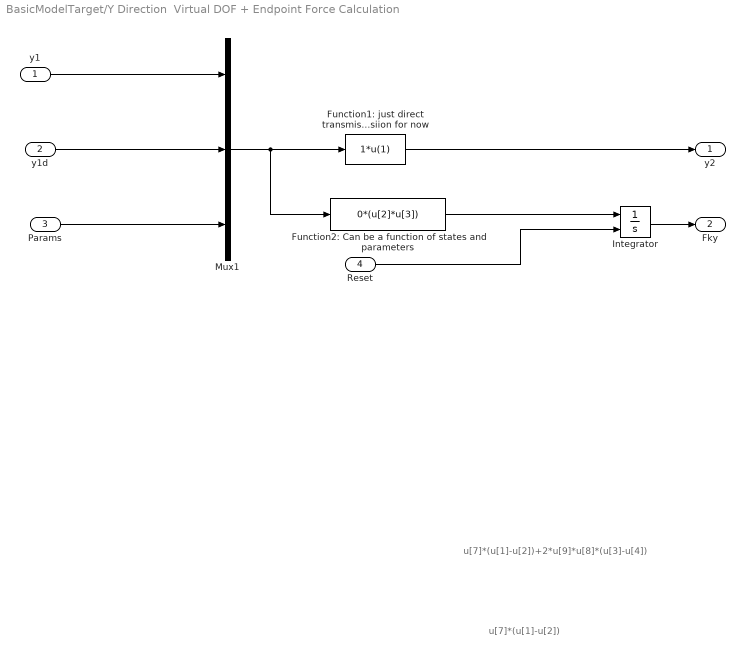
== system BasicModelTarget/Y Direction  Virtual DOF + Endpoint Force Calculation ==
  note: u[7]*(u[1]-u[2])+2*u[9]*u[8]*(u[3]-u[4])
  note: u[7]*(u[1]-u[2])
  y1 : Inport  OutDataType=sfix(16)  OutScaling=2^0
  y1d : Inport  Port=2  OutDataType=sfix(16)  OutScaling=2^0
  Params : Inport  Port=3  OutDataType=sfix(16)  OutScaling=2^0
  Reset : Inport  Port=4  OutDataType=sfix(16)  OutScaling=2^0
  Function1: just direct transmissiion for now : Fcn  Expr=1*u(1)
  Function2: Can be a function of states and parameters : Fcn  Expr=0*(u[2]*u[3])
  Integrator : Integrator  ExternalReset=either
  Mux1 : Mux  Inputs=3
  y2 : Outport  OutDataType=sfix(16)  OutScaling=2^0
  Fky : Outport  Port=2  OutDataType=sfix(16)  OutScaling=2^0
  wires:
  y1d/1 -> Mux1/2
  Params/1 -> Mux1/3
  Reset/1 -> Integrator/2
  Integrator/1 -> Fky/1
  Function2: Can be a function of states and parameters/1 -> Integrator/1
  y1/1 -> Mux1/1
  Mux1/1 -> Function1: just direct transmissiion for now/1, Function2: Can be a function of states and parameters/1
  Function1: just direct transmissiion for now/1 -> y2/1

== system BasicModelTarget/Manipulandum  Dynamic Compensation: will function poorly with unfiltered inputs/2x2Make ==
  In1 : Inport  OutDataType=sfix(16)  OutScaling=2^0
  In2 : Inport  Port=2  OutDataType=sfix(16)  OutScaling=2^0
  In3 : Inport  Port=3  OutDataType=sfix(16)  OutScaling=2^0
  In4 : Inport  Port=4  OutDataType=sfix(16)  OutScaling=2^0
  Add : Sum  Inputs=++++  OutDataType=sfix(16)  OutScaling=2^-10
  Gain : Gain  Gain=[1, 0; 0, 0]  ParameterDataType=sfix(16)  ParameterScaling=2^0  OutDataType=sfix(16)  OutScaling=2^0
  Gain1 : Gain  Gain=[0, 1; 0, 0]  ParameterDataType=sfix(16)  ParameterScaling=2^0  OutDataType=sfix(16)  OutScaling=2^0
  Gain2 : Gain  Gain=[0, 0; 1, 0]  ParameterDataType=sfix(16)  ParameterScaling=2^0  OutDataType=sfix(16)  OutScaling=2^0
  Gain3 : Gain  Gain=[0, 0; 0, 1]  ParameterDataType=sfix(16)  ParameterScaling=2^0  OutDataType=sfix(16)  OutScaling=2^0
  Out1 : Outport  OutDataType=sfix(16)  OutScaling=2^0
  wires:
  Add/1 -> Out1/1
  Gain/1 -> Add/1
  Gain1/1 -> Add/2
  Gain2/1 -> Add/3
  Gain3/1 -> Add/4
  In1/1 -> Gain/1
  In2/1 -> Gain1/1
  In3/1 -> Gain2/1
  In4/1 -> Gain3/1

== system BasicModelTarget/Manipulandum  Dynamic Compensation: will function poorly with unfiltered inputs/2x2Make1 ==
  In1 : Inport  OutDataType=sfix(16)  OutScaling=2^0
  In2 : Inport  Port=2  OutDataType=sfix(16)  OutScaling=2^0
  In3 : Inport  Port=3  OutDataType=sfix(16)  OutScaling=2^0
  In4 : Inport  Port=4  OutDataType=sfix(16)  OutScaling=2^0
  Add : Sum  Inputs=++++  OutDataType=sfix(16)  OutScaling=2^-10
  Gain : Gain  Gain=[1, 0; 0, 0]  ParameterDataType=sfix(16)  ParameterScaling=2^0  OutDataType=sfix(16)  OutScaling=2^0
  Gain1 : Gain  Gain=[0, 1; 0, 0]  ParameterDataType=sfix(16)  ParameterScaling=2^0  OutDataType=sfix(16)  OutScaling=2^0
  Gain2 : Gain  Gain=[0, 0; 1, 0]  ParameterDataType=sfix(16)  ParameterScaling=2^0  OutDataType=sfix(16)  OutScaling=2^0
  Gain3 : Gain  Gain=[0, 0; 0, 1]  ParameterDataType=sfix(16)  ParameterScaling=2^0  OutDataType=sfix(16)  OutScaling=2^0
  Out1 : Outport  OutDataType=sfix(16)  OutScaling=2^0
  wires:
  In4/1 -> Gain3/1
  In3/1 -> Gain2/1
  In2/1 -> Gain1/1
  In1/1 -> Gain/1
  Gain3/1 -> Add/4
  Gain2/1 -> Add/3
  Gain1/1 -> Add/2
  Gain/1 -> Add/1
  Add/1 -> Out1/1

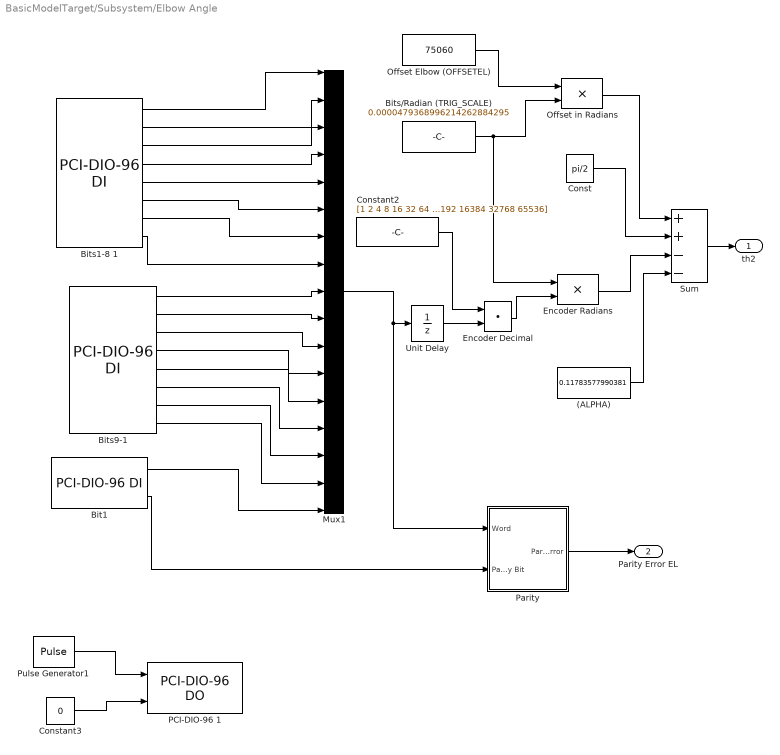
== system BasicModelTarget/Subsystem/Elbow Angle ==
  (ALPHA) : Constant  Description=Angle created by the offset of the elbow link from elbow joint  Value=0.11783577990381  OutDataType=sfix(16)  OutScaling=2^0
  Bit1 : xpcnilib/Digital Input/PCI-DIO-96 DI  channel=[1 4]  port=C  chip=3  sampletime=sp  slot=-1
  Bits/Radian (TRIG_SCALE) : Constant  Value=0.0000479368996214262884295  OutDataType=sfix(16)  OutScaling=2^0
  Bits1-8 1 : xpcnilib/Digital Input/PCI-DIO-96 DI  channel=[1 2 3 4 5 6 7 8]  port=A  chip=3  sampletime=sp  slot=-1
  Bits9-1 : xpcnilib/Digital Input/PCI-DIO-96 DI  channel=[ 1 2 3 4 5 6 7 8]  port=B  chip=3  sampletime=sp  slot=-1
  Const : Constant  Description=compensation for direction orientation  Value=pi/2  OutDataType=sfix(16)  OutScaling=2^0
  Constant2 : Constant  Value=[1 2 4 8 16 32 64 128 256 512 1024 2048 4096 8192 16384 32768 65536]  VectorParams1D=off  OutDataType=sfix(16)  OutScaling=2^0
  Constant3 : Constant  Value=0  VectorParams1D=off  OutDataType=sfix(16)  OutScaling=2^0
  Encoder Decimal : DotProduct  OutDataType=sfix(16)  OutScaling=2^-10  InputSameDT=on  OutDataTypeStr=Inherit: Inherit via internal rule
  Encoder Radians : Product  OutDataType=sfix(16)  OutScaling=2^0  SaturateOnIntegerOverflow=on  InputSameDT=on  OutDataTypeStr=Inherit: Same as first input
  Mux1 : Mux  Inputs=17
      settings: DisplayOption=signals
  "Offset Elbow (OFFSETEL) " : Constant  Value=75060  OutDataType=sfix(16)  OutScaling=2^0
  Offset in Radians : Product  OutDataType=sfix(16)  OutScaling=2^0  SaturateOnIntegerOverflow=on  InputSameDT=on  OutDataTypeStr=Inherit: Same as first input
  PCI-DIO-96 1 : xpcnilib/Digital Output/PCI-DIO-96 DO  channel=[1 2]  port=A  reset=[1]  initValue=[0]  chip=4  sampletime=-1  slot=-1
  Parity : Subsystem
  Pulse Generator1 : DiscretePulseGenerator  Amplitude=1  Period=2  PulseWidth=1  PhaseDelay=0  SampleTime=sp/2
  Sum : Sum  Inputs=++|--  OutDataType=sfix(16)  OutScaling=2^0  SaturateOnIntegerOverflow=on  InputSameDT=on  OutDataTypeStr=Inherit: Same as first input
  Unit Delay : UnitDelay  SampleTime=sp
  th2 : Outport  OutDataType=sfix(16)  OutScaling=2^0
  Parity Error EL : Outport  Port=2  OutDataType=sfix(16)  OutScaling=2^0
  wires:
  Bits1-8 1/1 -> Mux1/1
  Bits1-8 1/2 -> Mux1/2
  Bits1-8 1/3 -> Mux1/3
  Bits1-8 1/4 -> Mux1/4
  Bits1-8 1/5 -> Mux1/5
  Bits1-8 1/6 -> Mux1/6
  Bits1-8 1/7 -> Mux1/7
  Bits1-8 1/8 -> Mux1/8
  Bit1/1 -> Mux1/17
  Bits9-1/8 -> Mux1/16
  Bits9-1/6 -> Mux1/14
  Bits9-1/7 -> Mux1/15
  Bits9-1/5 -> Mux1/13
  Bits9-1/4 -> Mux1/12
  Bits9-1/3 -> Mux1/11
  Bits9-1/2 -> Mux1/10
  Bits9-1/1 -> Mux1/9
  Mux1/1 -> Parity/1("Word "), Unit Delay/1
  Constant3/1 -> PCI-DIO-96 1/2
  Pulse Generator1/1 -> PCI-DIO-96 1/1
  Bit1/2 -> Parity/2(Parity Bit)
  Parity/1(Parity Error) -> Parity Error EL/1
  Bits/Radian (TRIG_SCALE)/1 -> Offset in Radians/2, Encoder Radians/1
  "Offset Elbow (OFFSETEL) "/1 -> Offset in Radians/1
  Sum/1 -> th2/1
  Encoder Decimal/1 -> Encoder Radians/2
  Encoder Radians/1 -> Sum/3
  (ALPHA)/1 -> Sum/4
  Const/1 -> Sum/2
  Offset in Radians/1 -> Sum/1
  Constant2/1 -> Encoder Decimal/1
  Unit Delay/1 -> Encoder Decimal/2

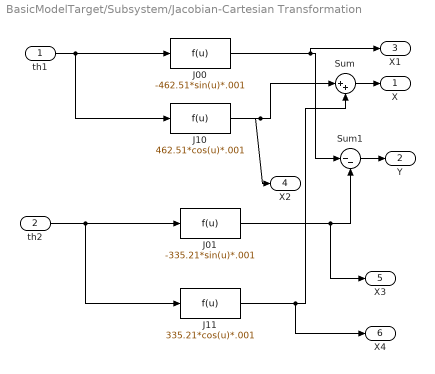
== system BasicModelTarget/Subsystem/Jacobian-Cartesian Transformation ==
  th1 : Inport  OutDataType=sfix(16)  OutScaling=2^0
  th2 : Inport  Port=2  OutDataType=sfix(16)  OutScaling=2^0
  J00 : Fcn  Expr=-462.51*sin(u)*.001
  J01 : Fcn  Expr=-335.21*sin(u)*.001
  J10 : Fcn  Expr=462.51*cos(u)*.001
  J11 : Fcn  Expr=335.21*cos(u)*.001
  Sum : Sum  Inputs=|++  OutDataType=sfix(16)  OutScaling=2^0  SaturateOnIntegerOverflow=on  InputSameDT=on  OutDataTypeStr=Inherit: Same as first input
  Sum1 : Sum  Inputs=|--  OutDataType=sfix(16)  OutScaling=2^0  SaturateOnIntegerOverflow=on  InputSameDT=on  OutDataTypeStr=Inherit: Same as first input
  X : Outport  OutDataType=sfix(16)  OutScaling=2^0
  Y : Outport  Port=2  OutDataType=sfix(16)  OutScaling=2^0
  X1 : Outport  Port=3  OutDataType=sfix(16)  OutScaling=2^0
  X2 : Outport  Port=4  OutDataType=sfix(16)  OutScaling=2^0
  X3 : Outport  Port=5  OutDataType=sfix(16)  OutScaling=2^0
  X4 : Outport  Port=6  OutDataType=sfix(16)  OutScaling=2^0
  wires:
  J10/1 -> Sum/1, X2/1
  J11/1 -> Sum/2, X4/1
  J01/1 -> Sum1/2, X3/1
  th1/1 -> J00/1, J10/1
  th2/1 -> J11/1, J01/1
  Sum/1 -> X/1
  Sum1/1 -> Y/1
  J00/1 -> Sum1/1, X1/1

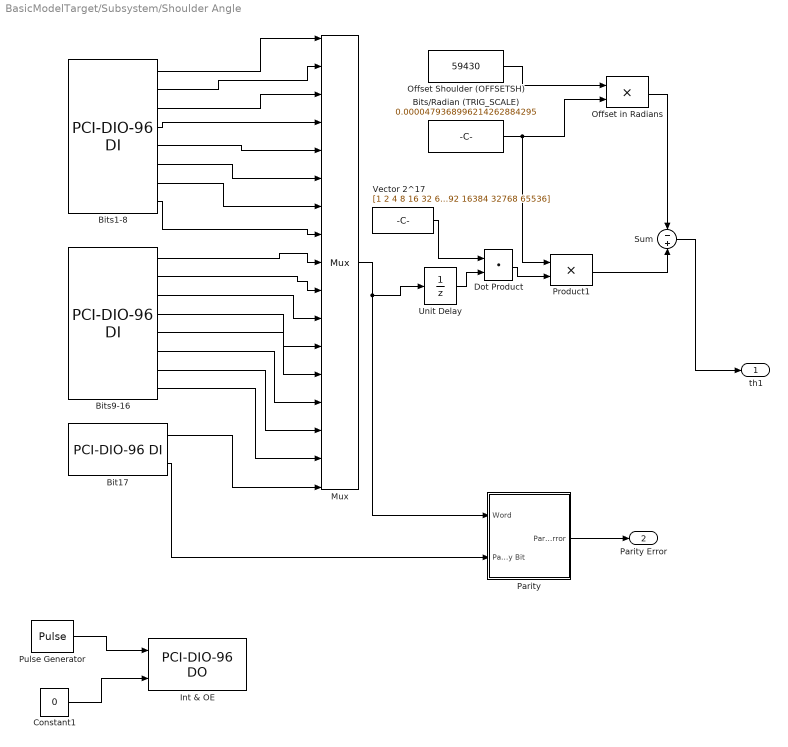
== system BasicModelTarget/Subsystem/Shoulder Angle ==
  Bit17 : xpcnilib/Digital Input/PCI-DIO-96 DI  channel=[1 4]  port=C  chip=1  sampletime=sp  slot=-1
  Bits/Radian (TRIG_SCALE) : Constant  Value=0.0000479368996214262884295  OutDataType=sfix(16)  OutScaling=2^0
  "Bits1-8 " : xpcnilib/Digital Input/PCI-DIO-96 DI  channel=[1 2 3 4 5 6 7 8]  port=A  chip=1  sampletime=sp  slot=-1
  Bits9-16 : xpcnilib/Digital Input/PCI-DIO-96 DI  channel=[ 1 2 3 4 5 6 7 8]  port=B  chip=1  sampletime=sp  slot=-1
  Constant1 : Constant  Value=0  OutDataType=sfix(16)  OutScaling=2^0
  Dot Product : DotProduct  OutDataType=sfix(16)  OutScaling=2^-10  InputSameDT=on  OutDataTypeStr=Inherit: Inherit via internal rule
  Int & OE : xpcnilib/Digital Output/PCI-DIO-96 DO  channel=[1 2]  port=A  reset=[1]  initValue=[0]  chip=2  sampletime=-1  slot=-1
  Mux : Mux  Inputs=17
      settings: DisplayOption=signals
  "Offset Shoulder (OFFSETSH) " : Constant  Value=59430  OutDataType=sfix(16)  OutScaling=2^0
  Offset in Radians : Product  OutDataType=sfix(16)  OutScaling=2^0  SaturateOnIntegerOverflow=on  InputSameDT=on  OutDataTypeStr=Inherit: Same as first input
  Parity : Subsystem
  Product1 : Product  OutDataType=sfix(16)  OutScaling=2^0  SaturateOnIntegerOverflow=on  InputSameDT=on  OutDataTypeStr=Inherit: Same as first input
  Pulse Generator : DiscretePulseGenerator  Amplitude=1  Period=2  PulseWidth=1  PhaseDelay=0  SampleTime=sp/2
  Sum : Sum  Inputs=-|+  OutDataType=sfix(16)  OutScaling=2^0  SaturateOnIntegerOverflow=on  InputSameDT=on  OutDataTypeStr=Inherit: Same as first input
  Unit Delay : UnitDelay  SampleTime=sp
  Vector 2^17 : Constant  Value=[1 2 4 8 16 32 64 128 256 512 1024 2048 4096 8192 16384 32768 65536]  VectorParams1D=off  OutDataType=sfix(16)  OutScaling=2^0
  th1 : Outport  OutDataType=sfix(16)  OutScaling=2^0
  Parity Error : Outport  Port=2  OutDataType=sfix(16)  OutScaling=2^0
  wires:
  "Bits1-8 "/1 -> Mux/1
  "Bits1-8 "/2 -> Mux/2
  "Bits1-8 "/3 -> Mux/3
  "Bits1-8 "/4 -> Mux/4
  "Bits1-8 "/5 -> Mux/5
  "Bits1-8 "/6 -> Mux/6
  "Bits1-8 "/7 -> Mux/7
  "Bits1-8 "/8 -> Mux/8
  Bit17/1 -> Mux/17
  Bits9-16/8 -> Mux/16
  Bits9-16/6 -> Mux/14
  Bits9-16/7 -> Mux/15
  Bits9-16/5 -> Mux/13
  Bits9-16/4 -> Mux/12
  Bits9-16/3 -> Mux/11
  Bits9-16/2 -> Mux/10
  Bits9-16/1 -> Mux/9
  Mux/1 -> Parity/1("Word "), Unit Delay/1
  Parity/1(Parity Error) -> Parity Error/1
  Bits/Radian (TRIG_SCALE)/1 -> Offset in Radians/2, Product1/1
  "Offset Shoulder (OFFSETSH) "/1 -> Offset in Radians/1
  Dot Product/1 -> Product1/2
  Product1/1 -> Sum/2
  Offset in Radians/1 -> Sum/1
  Sum/1 -> th1/1
  Bit17/2 -> Parity/2(Parity Bit)
  Pulse Generator/1 -> Int & OE/1
  Constant1/1 -> Int & OE/2
  Vector 2^17/1 -> Dot Product/1
  Unit Delay/1 -> Dot Product/2

== system BasicModelTarget/Subsystem/Elbow Angle/Parity ==
  "Word " : Inport  OutDataType=sfix(16)  OutScaling=2^0
  Parity Bit : Inport  Port=2  OutDataType=sfix(16)  OutScaling=2^0
  Constant : Constant  Value=2  OutDataType=sfix(16)  OutScaling=2^0
  Demux : Demux  Outputs=17
  Math Function : Math  Operator=mod  OutDataType=sfix(16)  OutScaling=2^0  SaturateOnIntegerOverflow=on
  Sum : Sum  Inputs=|++++++++++++++++++  OutDataType=sfix(16)  OutScaling=2^0  SaturateOnIntegerOverflow=on  InputSameDT=on  OutDataTypeStr=Inherit: Same as first input
  Parity Error : Outport  OutDataType=sfix(16)  OutScaling=2^0
  wires:
  Math Function/1 -> Parity Error/1
  Constant/1 -> Math Function/2
  Sum/1 -> Math Function/1
  Parity Bit/1 -> Sum/18
  "Word "/1 -> Demux/1
  Demux/17 -> Sum/17
  Demux/16 -> Sum/16
  Demux/15 -> Sum/15
  Demux/14 -> Sum/14
  Demux/13 -> Sum/13
  Demux/12 -> Sum/12
  Demux/11 -> Sum/11
  Demux/10 -> Sum/10
  Demux/9 -> Sum/9
  Demux/8 -> Sum/8
  Demux/7 -> Sum/7
  Demux/6 -> Sum/6
  Demux/5 -> Sum/5
  Demux/4 -> Sum/4
  Demux/3 -> Sum/3
  Demux/2 -> Sum/2
  Demux/1 -> Sum/1

== system BasicModelTarget/Subsystem/Shoulder Angle/Parity ==
  "Word " : Inport  OutDataType=sfix(16)  OutScaling=2^0
  Parity Bit : Inport  Port=2  OutDataType=sfix(16)  OutScaling=2^0
  Constant : Constant  Value=2  OutDataType=sfix(16)  OutScaling=2^0
  Demux : Demux  Outputs=17
  Math Function : Math  Operator=mod  OutDataType=sfix(16)  OutScaling=2^0  SaturateOnIntegerOverflow=on
  Sum : Sum  Inputs=|++++++++++++++++++  OutDataType=sfix(16)  OutScaling=2^0  SaturateOnIntegerOverflow=on  InputSameDT=on  OutDataTypeStr=Inherit: Same as first input
  Parity Error : Outport  OutDataType=sfix(16)  OutScaling=2^0
  wires:
  Math Function/1 -> Parity Error/1
  Constant/1 -> Math Function/2
  Sum/1 -> Math Function/1
  Parity Bit/1 -> Sum/18
  "Word "/1 -> Demux/1
  Demux/17 -> Sum/17
  Demux/16 -> Sum/16
  Demux/15 -> Sum/15
  Demux/14 -> Sum/14
  Demux/13 -> Sum/13
  Demux/12 -> Sum/12
  Demux/11 -> Sum/11
  Demux/10 -> Sum/10
  Demux/9 -> Sum/9
  Demux/8 -> Sum/8
  Demux/7 -> Sum/7
  Demux/6 -> Sum/6
  Demux/5 -> Sum/5
  Demux/4 -> Sum/4
  Demux/3 -> Sum/3
  Demux/2 -> Sum/2
  Demux/1 -> Sum/1
